simulink subsystem "modulador_tension_trif"  (R2020a)
settings: Solver=VariableStepAuto  StartTime=0.0  StopTime=10.0  RelTol=1e-3
settings Model: Creator=Ferran  LastModifiedBy=Ferran

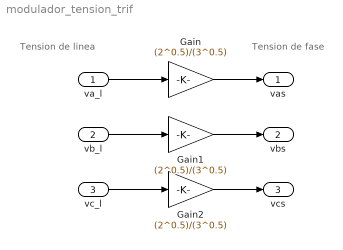
== system modulador_tension_trif ==
  note: Tension de linea
  note: Tension de fase
  va_l : Inport
  vb_l : Inport  Port=2
  vc_l : Inport  Port=3
  Gain : Gain  Gain=(2^0.5)/(3^0.5)
  Gain1 : Gain  Gain=(2^0.5)/(3^0.5)
  Gain2 : Gain  Gain=(2^0.5)/(3^0.5)
  vas : Outport
  vbs : Outport  Port=2
  vcs : Outport  Port=3
  wires:
  va_l/1 -> Gain/1
  Gain/1 -> vas/1
  vc_l/1 -> Gain2/1
  Gain2/1 -> vcs/1
  vb_l/1 -> Gain1/1
  Gain1/1 -> vbs/1
